simulink model "normal"  (R2015a)
settings: Solver=ode45  StartTime=0.0  StopTime=10.0  RelTol=1e-3
values from neighbouring files (symbols this model uses):
  K = lqr(A, B, Qr, Rr)    [LabCEE.m]    (also in fp_ini.m)
  L = lqe(A, G, C, Qe, Re)    [LabCEE.m]    (also in fp_ini.m)
  MOTOR_SAT = 5    [fp_ini.m]
  TH1_BOUND = 120*pi/180    (= 2.09439510239)    [fp_ini.m]
  TH2_BOUND = 30*pi/180    (= 0.523598775598)    [fp_ini.m]
  TIME_DELAY = 6    [fp_ini.m]
undefined symbols (not defined in the file or in its folder): A, B, C, National_Instruments, PCI
libraries: sldrtlib x3
settings Model: Creator=Alunos  LastModifiedBy=Alunos

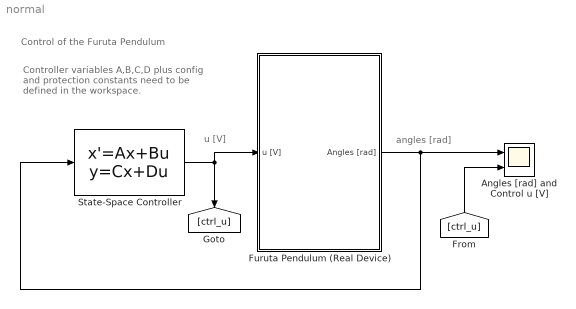
== system normal ==
  note: angles [rad]
  note: u [V]
  note: Controller variables A,B,C,D
      | plus config and protection constants
      | need to be defined in the workspace.
  note: Control of the Furuta Pendulum
  Angles [rad] and Control u [V] : Scope  NumInputPorts=2
      settings: YMin=-0.3~-2.5  YMax=0.15~2.5  SaveName=pendulum  SampleInput=on
  Furuta Pendulum (Real Device) : Subsystem
      mask Display: image('fp_pict.jpg')
  State-Space Controller : StateSpace  A=A-B*K-L*C  B=L  C=-K  D=D'  X0=0
  wires:
  State-Space Controller/1 -> Furuta Pendulum (Real Device)/1(u [V]), [ctrl_u]
  [ctrl_u] -> Angles [rad] and Control u [V]/2
  Furuta Pendulum (Real Device)/1(Angles [rad]) -> State-Space Controller/1, Angles [rad] and Control u [V]/1

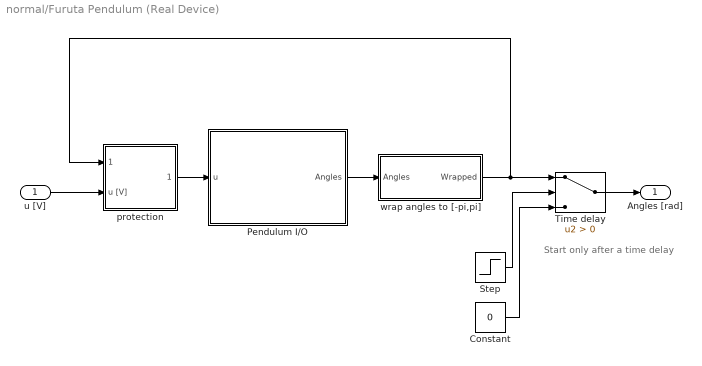
== system normal/Furuta Pendulum (Real Device) ==
  note: Start only after
      | a time delay
  u [V] : Inport
  Constant : Constant  Value=0
  Pendulum I/O : Subsystem
  Step : Step  Time=TIME_DELAY  SampleTime=0
  Time delay : Switch  Criteria=u2 > Threshold
  protection : Subsystem
  wrap angles to [-pi,pi] : Subsystem
  Angles [rad] : Outport
  wires:
  Pendulum I/O/1(Angles) -> wrap angles to [-pi,pi]/1(Angles)
  protection/1(u_out [V]) -> Pendulum I/O/1(u)
  Step/1 -> Time delay/2
  Constant/1 -> Time delay/3
  Time delay/1 -> Angles [rad]/1
  wrap angles to [-pi,pi]/1(Wrapped) -> Time delay/1, protection/1(angles [rad])
  u [V]/1 -> protection/2(u [V])

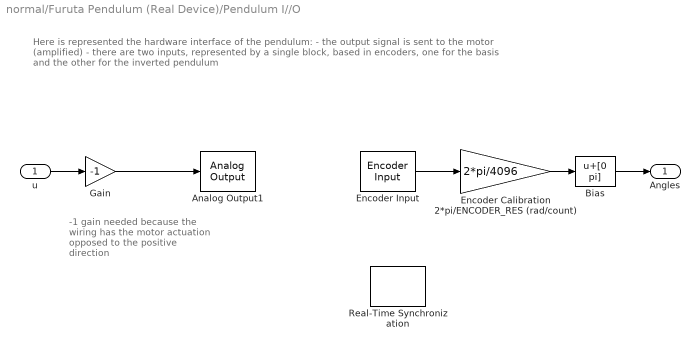
== system normal/Furuta Pendulum (Real Device)/Pendulum I//O ==
  note: Here is represented the hardware interface of the pendulum:
      | - the output signal is sent to the motor (amplified)
      | - there are two inputs, represented by a single block, based in encoders,
      | one for the basis and the other for the inverted pendulum
  note: -1 gain needed
      | because the wiring
      | has the motor
      | actuation opposed to
      | the positive direction
  u : Inport
  Analog Output1 : sldrtlib/Analog Output  SampleTime=0.001  MaxMissedTicks=inf  ShowMissedTicks=off  YieldWhenWaiting=off  DrvName=National_Instruments/PCI-6221  DrvAddress=4294967295  DrvOptions=[0 0 0 2 2]  Channels=1  RangeMode=1  VoltRange=1  InitialValue=[]  FinalValue=0
      settings: AttributesFormatString=National Instruments\nPCI-6221 [auto]
  Bias : Bias  Bias=[0 pi]
  Encoder Calibration 2*pi/ENCODER_RES (rad/count) : Gain  Gain=2*pi/4096  SaturateOnIntegerOverflow=on  OutDataTypeStr=Inherit: Same as input  ParamDataTypeStr=Inherit: Same as input
  Encoder Input : sldrtlib/Encoder Input  SampleTime=0.001  MaxMissedTicks=inf  ShowMissedTicks=off  YieldWhenWaiting=off  DrvName=National_Instruments/PCI-6221  DrvAddress=4294967295  DrvOptions=[0 0 0 2 2]  Channels=1:2  QuadMode=3  IndexPulse=2  InputFilter=Inf  DataType=1
      settings: AttributesFormatString=National Instruments\nPCI-6221 [auto]
  Gain : Gain  Gain=-1
  Real-Time Synchronization : sldrtlib/Real-Time Synchronization  SampleTime=0.001  MaxMissedTicks=inf  ShowMissedTicks=off  YieldWhenWaiting=off
  Angles : Outport
  wires:
  u/1 -> Gain/1
  Encoder Calibration 2*pi/ENCODER_RES (rad/count)/1 -> Bias/1
  Encoder Input/1 -> Encoder Calibration 2*pi/ENCODER_RES (rad/count)/1
  Bias/1 -> Angles/1
  Gain/1 -> Analog Output1/1

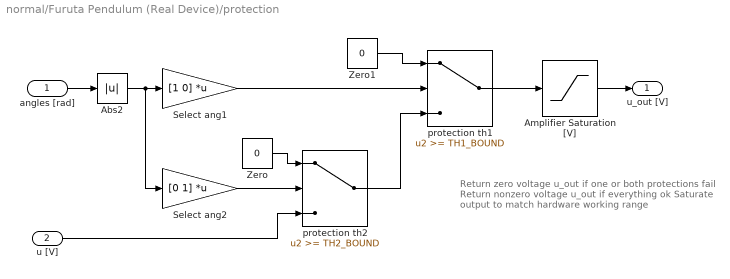
== system normal/Furuta Pendulum (Real Device)/protection ==
  note: Return zero voltage u_out
      | if one or both protections fail
      |
      | Return nonzero voltage u_out
      | if everything ok
      |
      | Saturate output to match hardware
      | working range
  angles [rad] : Inport
  u [V] : Inport  Port=2
  Abs2 : Abs
  Amplifier Saturation [V] : Saturate  UpperLimit=MOTOR_SAT  LowerLimit=-MOTOR_SAT
  Select ang1 : Gain  Gain=[1 0]  Multiplication=Matrix(K*u)
  Select ang2 : Gain  Gain=[0 1]  Multiplication=Matrix(K*u)
  Zero : Constant  Value=0
  Zero1 : Constant  Value=0
  protection th1 : Switch  Threshold=TH1_BOUND
  protection th2 : Switch  Threshold=TH2_BOUND
  u_out [V] : Outport
  wires:
  Zero/1 -> protection th2/1
  protection th1/1 -> Amplifier Saturation [V]/1
  Amplifier Saturation [V]/1 -> u_out [V]/1
  Abs2/1 -> Select ang2/1, Select ang1/1
  Select ang1/1 -> protection th1/2
  u [V]/1 -> protection th2/3
  protection th2/1 -> protection th1/3
  Select ang2/1 -> protection th2/2
  Zero1/1 -> protection th1/1
  angles [rad]/1 -> Abs2/1

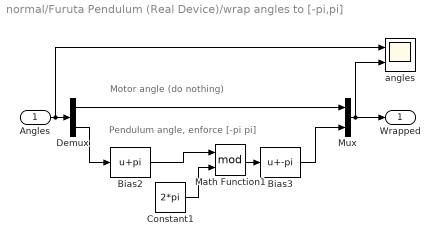
== system normal/Furuta Pendulum (Real Device)/wrap angles to [-pi,pi] ==
  note: Pendulum angle, enforce [-pi pi]
  note: Motor angle (do nothing)
  Angles : Inport
  Bias2 : Bias  Bias=pi
  Bias3 : Bias  Bias=-pi
  Constant1 : Constant  Value=2*pi
  Demux : Demux  Outputs=2
  Math Function1 : Math  Operator=mod  SaturateOnIntegerOverflow=on
  Mux : Mux  Inputs=2
  angles : Scope  NumInputPorts=2
      settings: YMin=-1~-4  YMax=7~4
  Wrapped : Outport
  wires:
  Bias2/1 -> Math Function1/1
  Constant1/1 -> Math Function1/2
  Math Function1/1 -> Bias3/1
  Angles/1 -> angles/1, Demux/1
  Demux/1 -> Mux/1
  Mux/1 -> angles/2, Wrapped/1
  Bias3/1 -> Mux/2
  Demux/2 -> Bias2/1
